simulink model "PIDTuning_obtencion"  (R2023b)
settings: Solver=VariableStepAuto  StartTime=0.0  StopTime=2  FixedStep=0.01  RelTol=1e-3
undefined symbols (not defined in the file or in its folder): delay, K, tau
settings Model: Creator=SaulCM  LastModifiedBy=saulc
settings DebuggingCC: UnconnectedInputMsg=warning  UnconnectedOutputMsg=warning  UnconnectedLineMsg=warning
settings ModelReferenceCC: EnableRefExpFcnMdlSchedulingChecks=on
settings RTWCC: DLArmComputeVersion=19.05

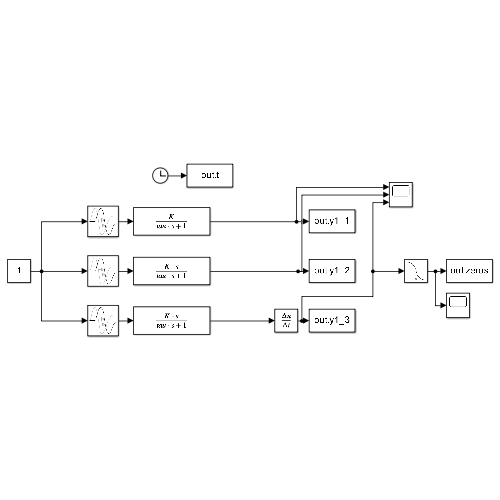
[thumbnail: Simulink's stored preview of the top-level diagram]
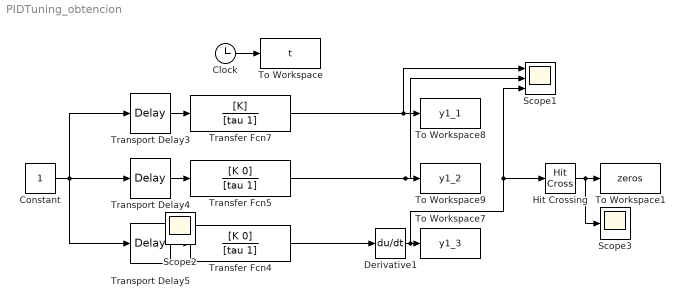
== system PIDTuning_obtencion ==
  Clock : Clock
  Constant : Constant
  Derivative1 : Derivative
  Hit Crossing : HitCross  HitCrossingDirection=falling
  Scope1 : Scope  NumInputPorts=3
  Scope3 : Scope
  To Workspace : ToWorkspace  VariableName=t  SampleTime=0.001
      settings: Save2DSignal=2-D array (concatenate along first dimension)
  To Workspace1 : ToWorkspace  VariableName=zeros  SampleTime=0.001
      settings: Save2DSignal=2-D array (concatenate along first dimension)
  To Workspace7 : ToWorkspace  VariableName=y1_3  SampleTime=0.001
      settings: Save2DSignal=2-D array (concatenate along first dimension)
  To Workspace8 : ToWorkspace  VariableName=y1_1  SampleTime=0.001
      settings: Save2DSignal=2-D array (concatenate along first dimension)
  To Workspace9 : ToWorkspace  VariableName=y1_2  SampleTime=0.001
      settings: Save2DSignal=2-D array (concatenate along first dimension)
  Transfer Fcn4 : TransferFcn  Numerator=[K 0]  Denominator=[tau 1]
  Transfer Fcn5 : TransferFcn  Numerator=[K 0]  Denominator=[tau 1]
  Transfer Fcn7 : TransferFcn  Numerator=[K]  Denominator=[tau 1]
  Transport Delay3 : TransportDelay  DelayTime=delay
  Transport Delay4 : TransportDelay  DelayTime=delay
  Transport Delay5 : TransportDelay  DelayTime=delay
  Scope2 : Scope
  wires:
  Constant/1 -> Transport Delay5/1, Transport Delay4/1, Transport Delay3/1
  Clock/1 -> To Workspace/1
  Derivative1/1 -> Hit Crossing/1, Scope1/3, To Workspace7/1
  Transfer Fcn4/1 -> Derivative1/1
  Transport Delay3/1 -> Transfer Fcn7/1
  Transfer Fcn7/1 -> Scope1/1, To Workspace8/1
  Transport Delay4/1 -> Transfer Fcn5/1
  Transport Delay5/1 -> Transfer Fcn4/1
  Transfer Fcn5/1 -> Scope1/2, To Workspace9/1
  Hit Crossing/1 -> Scope3/1, To Workspace1/1
